simulink model "hit_crossing_block"  (R2021a)
settings: Solver=VariableStepAuto  StartTime=0.0  StopTime=10.0  RelTol=1e-3
settings Model: Creator=DELL  LastModifiedBy=DELL

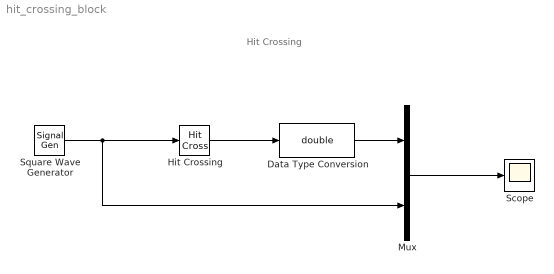
== system hit_crossing_block ==
  note: Hit Crossing
  Data Type Conversion : DataTypeConversion  OutDataTypeStr=double
  Hit Crossing : HitCross  HitCrossingOffset=2
  Mux : Mux  Inputs=2
  Scope : Scope
  Square Wave Generator : SignalGenerator  WaveForm=square  Amplitude=5  Frequency=.5  Units=rad/sec
  wires:
  Square Wave Generator/1 -> Mux/2, Hit Crossing/1
  Mux/1 -> Scope/1
  Hit Crossing/1 -> Data Type Conversion/1
  Data Type Conversion/1 -> Mux/1
